simulink model "est_model"  (R2023a)
settings: Solver=VariableStepAuto  StartTime=0.0  StopTime=0.1  FixedStep=Ts  RelTol=1e-6  AbsTol=1e-6
InitFcn:
  | est_model_paras
values from neighbouring files (symbols this model uses):
  Id = 0    [est_model_paras.m]
  Iq = 100    [est_model_paras.m]
  ki = [ki1 ki2]    [est_model_paras.m]    (also in svc_go_init.m = 2.96*Rs/sqrt(2)/N/Ts)
  kid_i = 3*Rs./Npi/Ts/Lq/Iq    [est_model_paras.m]
  kid_p = 3*Lq./Npi/Ts/Lq/Iq    [est_model_paras.m]
  kp = (3*Ld./N/Ts-Rs)/Lq/Iq    [est_model_paras.m]    (also in svc_go_init.m = -0.01944)
  kpi_i = 3*Rs./Npi/Ts    [est_model_paras.m]
  kpi_p = 3*Lq./Npi/Ts    [est_model_paras.m]
  Ld = 0.000891    [est_model_paras.m]    (also in svc_go_init.m = 0.00026)
  Lq = 0.000891    [est_model_paras.m]    (also in svc_go_init.m = 0.000636)
  phi_r = 0.012    [est_model_paras.m]    (also in svc_go_init.m = 0.078)
  Rs = 0.503    [est_model_paras.m]    (also in svc_go_init.m = 0.021)
  Ts = 1/8000    (= 0.000125)    [est_model_paras.m]    (also in svc_go_init.m)
  We = 2*pi*100    (= 628.318530718)    [est_model_paras.m]    (also in svc_go_init.m)
undefined symbols (not defined in the file or in its folder): DiscIntNeverNeededParam, ts
libraries: slpidlib x3
settings Model: Creator=LG-PC  LastModifiedBy=洲
settings SolverCC: AlgebraicLoopSolver=LineSearch
settings DataIOCC: ReturnWorkspaceOutputs=off
settings DebuggingCC: UnconnectedInputMsg=warning  UnconnectedOutputMsg=warning  UnconnectedLineMsg=warning  ArithmeticOperatorsInVariantConditions=warning
settings ModelReferenceCC: EnableRefExpFcnMdlSchedulingChecks=on
settings SFSimCC: SimUseLocalCustomCode=off  CustomCodeUndefinedFunction=UseInterfaceOnly
settings RTWCC: RTWUseLocalCustomCode=off

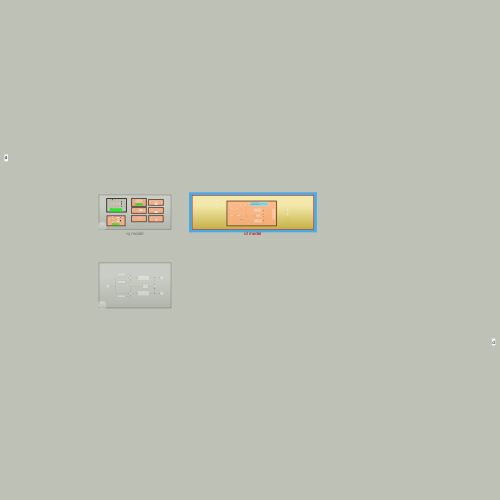
[thumbnail: Simulink's stored preview of the top-level diagram]
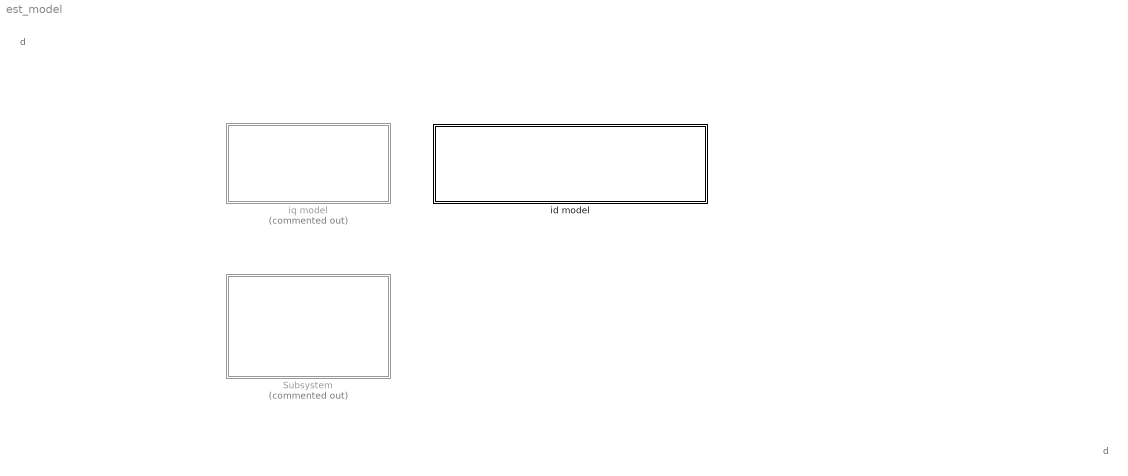
== system est_model ==
  note: d
  note: d
  Subsystem : Subsystem  Commented=on
  id model : Subsystem
  iq model : Subsystem  Commented=on

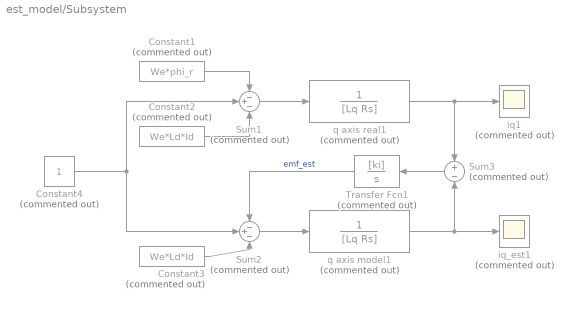
== system est_model/Subsystem ==
  Constant1 : Constant  Commented=on  Value=We*phi_r
  Constant2 : Constant  Commented=on  Value=We*Ld*Id
  Constant3 : Constant  Commented=on  Value=We*Ld*Id
  Constant4 : Constant  Commented=on
  Sum1 : Sum  Commented=on  Inputs=-+-
  Sum2 : Sum  Commented=on  Inputs=-+-
  Sum3 : Sum  Commented=on  Inputs=+-
  Transfer Fcn1 : TransferFcn  Commented=on  Numerator=[ki]  Denominator=[1 0]
  iq1 : Scope  Commented=on
  iq_est1 : Scope  Commented=on
  q axis model1 : TransferFcn  Commented=on  Denominator=[Lq Rs]
  q axis real1 : TransferFcn  Commented=on  Denominator=[Lq Rs]
  wires:
  q axis model1/1 -> iq_est1/1, Sum3/2
  Constant1/1 -> Sum1/1
  q axis real1/1 -> iq1/1, Sum3/1
  Sum3/1 -> Transfer Fcn1/1
  Constant3/1 -> Sum2/3
  Sum2/1 -> q axis model1/1
  Transfer Fcn1/1 -> Sum2/1  "emf_est"
  Constant2/1 -> Sum1/3
  Constant4/1 -> Sum1/2, Sum2/2
  Sum1/1 -> q axis real1/1

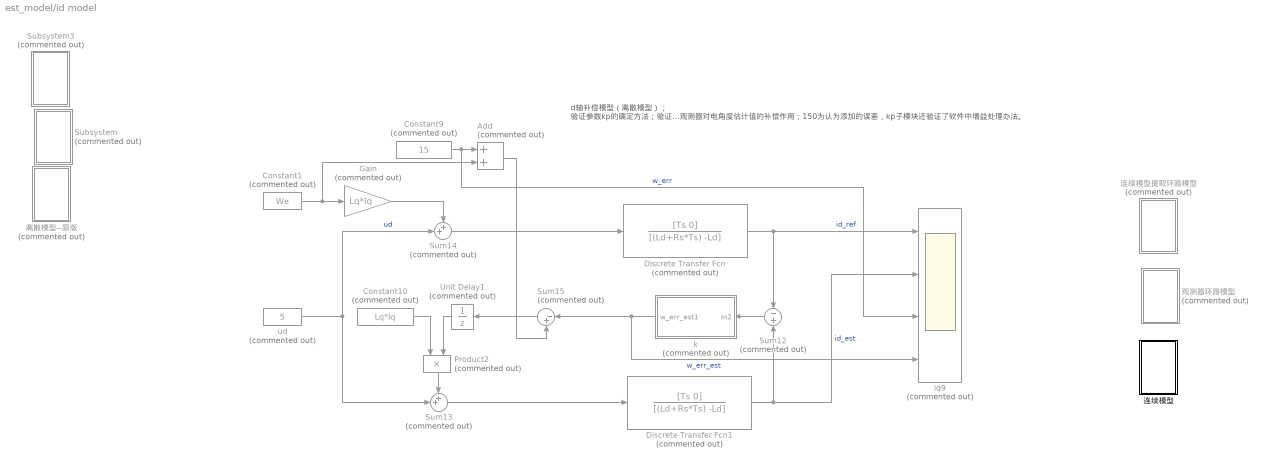
== system est_model/id model ==
  note: d轴补偿模型（离散模型）；
      | 验证参数kp的确定方法；验证观测器对电角度估计值的补偿作用；150为认为添加的误差，kp子模块还验证了软件中增益处理办法。
  Add : Sum  Commented=on
  Constant1 : Constant  Commented=on  Value=We
  Constant10 : Constant  Commented=on  Value=Lq*Iq
  Constant9 : Constant  Commented=on  Value=15
  Discrete Transfer Fcn : DiscreteTransferFcn  Commented=on  Numerator=[Ts 0]  Denominator=[(Ld+Rs*Ts) -Ld]
  Discrete Transfer Fcn1 : DiscreteTransferFcn  Commented=on  Numerator=[Ts 0]  Denominator=[(Ld+Rs*Ts) -Ld]
  Gain : Gain  Commented=on  Gain=Lq*Iq
  Product2 : Product  Commented=on
  Subsystem : Subsystem  Commented=on
  Subsystem3 : Subsystem  Commented=on
  Sum12 : Sum  Commented=on  Inputs=-+
  Sum13 : Sum  Commented=on  Inputs=++|
  Sum14 : Sum  Commented=on  Inputs=++|
  Sum15 : Sum  Commented=on  Inputs=|-+
  Unit Delay1 : UnitDelay  Commented=on  SampleTime=-1  HasFrameUpgradeWarning=on
  iq9 : Scope  Commented=on  NumInputPorts=4
  k : Subsystem  Commented=on
  ud : Constant  Commented=on  Value=5
  离散模型--原版 : Subsystem  Commented=on
  观测器环路模型 : Subsystem  Commented=on
  连续模型 : Subsystem
  连续模型提取环路模型 : Subsystem  Commented=on
  wires:
  ud/1 -> Sum13/2, Sum14/2  "ud"
  Add/1 -> Sum15/2
  Discrete Transfer Fcn/1 -> Sum12/1, iq9/1  "id_ref"
  Sum14/1 -> Discrete Transfer Fcn/1
  Sum15/1 -> Unit Delay1/1
  Product2/1 -> Sum13/1
  Discrete Transfer Fcn1/1 -> iq9/2, Sum12/2  "id_est"
  Unit Delay1/1 -> Product2/2
  Constant10/1 -> Product2/1
  Constant1/1 -> Add/2, Gain/1
  Gain/1 -> Sum14/1
  Sum13/1 -> Discrete Transfer Fcn1/1
  Constant9/1 -> iq9/3, Add/1  "w_err"
  k/1(w_err_est1) -> iq9/4, Sum15/1  "w_err_est"
  Sum12/1 -> k/1(In2)

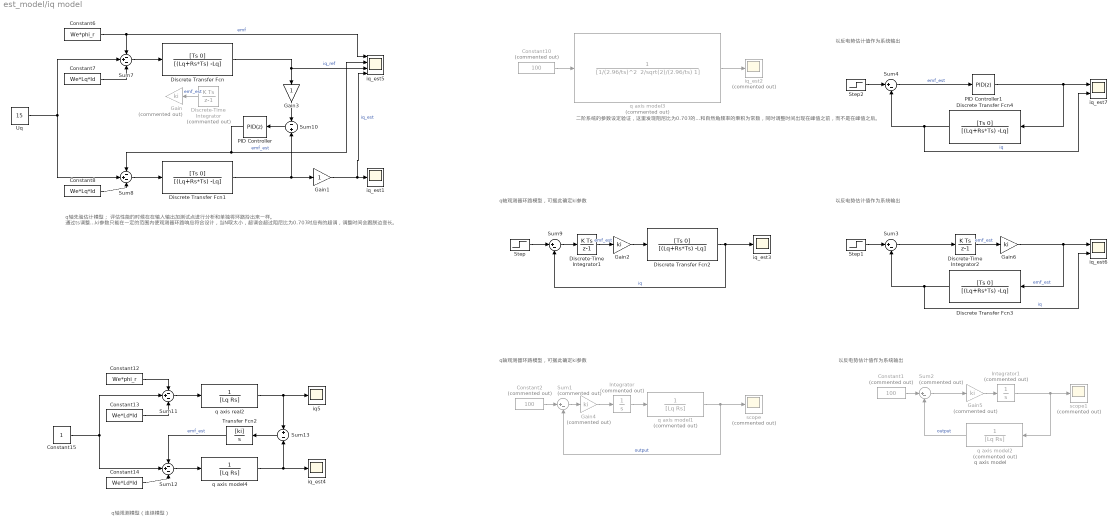
== system est_model/iq model ==
  note: q axis model
  note: q轴观测器环路模型，可据此确定ki参数
  note: 二阶系统的参数设定验证，这里发现阻尼比为0.707的时候，调整时间和自然角频率的乘积为常数，同时调整时间出现在峰值之前，而不是在峰值之后。
  note: q轴观测模型（连续模型）
  note: q轴先验估计模型；
      | 评估性能的时候在在输入输出加测试点进行分析和单独将环路拎出来一样。
      | 通过ts调整ki参数只能在一定的范围内使观测器环路响应符合设计，当N取太小，超调会超过阻尼比为0.707时应有的超调，调整时间会跟朕边变长。
  note: q轴观测器环路模型，可据此确定ki参数
  note: 以反电势估计值作为系统输出
  note: 以反电势估计值作为系统输出
  note: 以反电势估计值作为系统输出
  Constant1 : Constant  Commented=on  Value=100
  Constant10 : Constant  Commented=on  Value=100
  Constant12 : Constant  Value=We*phi_r
  Constant13 : Constant  Value=We*Ld*Id
  Constant14 : Constant  Value=We*Ld*Id
  Constant15 : Constant
  Constant2 : Constant  Commented=on  Value=100
  Constant6 : Constant  Value=We*phi_r
  Constant7 : Constant  Value=We*Lq*Id
  Constant8 : Constant  Value=We*Lq*Id
  Discrete Transfer Fcn{,1..4} (5 alike) : DiscreteTransferFcn  Numerator=[Ts 0]  Denominator=[(Lq+Rs*Ts) -Lq]
  Discrete-Time Integrator : DiscreteIntegrator  Commented=on  SampleTime=-1  ICPrevOutput=DiscIntNeverNeededParam  ICPrevScaledInput=DiscIntNeverNeededParam
  Discrete-Time Integrator1 : DiscreteIntegrator  SampleTime=-1  ICPrevOutput=DiscIntNeverNeededParam  ICPrevScaledInput=DiscIntNeverNeededParam
  Discrete-Time Integrator2 : DiscreteIntegrator  SampleTime=-1  ICPrevOutput=DiscIntNeverNeededParam  ICPrevScaledInput=DiscIntNeverNeededParam
  Gain : Gain  Commented=on  Gain=ki
  Gain1 : Gain
  Gain2 : Gain  Gain=ki
  Gain3 : Gain
  Gain4 : Gain  Commented=on  Gain=ki
  Gain5 : Gain  Commented=on  Gain=ki
  Gain6 : Gain  Gain=ki
  Integrator : Integrator  Commented=on
  Integrator1 : Integrator  Commented=on
  PID Controller : slpidlib/PID Controller  Controller=PID  Form=Parallel  TimeDomain=Discrete-time  UseExternalTs=off  SampleTime=-1  IntegratorMethod=Forward Euler  FilterMethod=Forward Euler  ControllerParametersSource=internal  P=kpi_p  I=kpi_i  UseKiTs=off  D=0  N=100  UseFilter=on  TunerSelectOption=Transfer Function Based (PID Tuner App)  InitialConditionSource=internal  InitialConditionForIntegrator=0  InitialConditionForFilter=0  DifferentiatorICPrevScaledInput=0  ExternalReset=none  TrackingMode=off  Kt=1  LimitOutput=off  SatLimitsSource=internal  UpperSaturationLimit=inf  LowerSaturationLimit=-inf  LinearizeAsGain=on  AntiWindupMode=none  Kb=1  LimitIntegrator=off  UpperIntegratorSaturationLimit=inf  LowerIntegratorSaturationLimit=-inf  POutMin=[]  POutMax=[]  IOutMin=[]  IOutMax=[]  DOutMin=[]  DOutMax=[]  NOutMin=[]  NOutMax=[]  SumOutMin=[]  SumOutMax=[]  SaturationOutMin=[]  SaturationOutMax=[]  PParamMin=[]  PParamMax=[]  IParamMin=[]  IParamMax=[]  DParamMin=[]  DParamMax=[]  NParamMin=[]  NParamMax=[]  KbParamMin=[]  KbParamMax=[]  KtParamMin=[]  KtParamMax=[]  KbOutMin=[]  KbOutMax=[]  KtOutMin=[]  KtOutMax=[]  IntegratorOutMin=[]  IntegratorOutMax=[]  FilterOutMin=[]  FilterOutMax=[]  SumI1OutMin=[]  SumI1OutMax=[]  SumI2OutMin=[]  SumI2OutMax=[]  SumI3OutMin=[]  SumI3OutMax=[]  SumI4OutMin=[]  SumI4OutMax=[]  SumDOutMin=[]  SumDOutMax=[]  DifferentiatorOutMin=[]  DifferentiatorOutMax=[]  FilterDiffOutCoefMin=[]  FilterDiffOutCoefMax=[]  ReciprocalOutMin=[]  ReciprocalOutMax=[]  SumDenOutMin=[]  SumDenOutMax=[]  SumNumOutMin=[]  SumNumOutMax=[]  DivideOutMin=[]  DivideOutMax=[]  UdiffTsProdOutMin=[]  UdiffTsProdOutMax=[]  NTsProdOutMin=[]  NTsProdOutMax=[]  UintegralTsProdOutMin=[]  UintegralTsProdOutMax=[]  UngainTsProdOutMin=[]  UngainTsProdOutMax=[]  ClampingZeroOutDataTypeStr=Inherit: Inherit via back propagation  ClampingZeroOutMin=[]  ClampingZeroOutMax=[]  FilterDenConstantOutDataTypeStr=Inherit: Inherit via back propagation  FilterDenConstantOutMin=[]  FilterDenConstantOutMax=[]  PCopyOutDataTypeStr=Inherit: Inherit via back propagation  PCopyOutMin=[]  PCopyOutMax=[]  NCopyOutDataTypeStr=Inherit: Inherit via back propagation  NCopyOutMin=[]  NCopyOutMax=[]  IntegratorContinuousStateAttributes=''  IntegratorStateMustResolveToSignalObject=off  IntegratorRTWStateStorageClass=Auto  FilterContinuousStateAttributes=''  FilterStateMustResolveToSignalObject=off  FilterRTWStateStorageClass=Auto  ParallelPVariant=InternalParameters  IdealPVariant=Disabled  IVariant=InternalParameters  DVariant=InternalParameters  IntegratorVariant=Discrete  SatVariant=Disabled  AWVariant=Passthrough  PCopyVariant=Disabled  TRVariant=Disabled  FdbkBlocksVariant=Forward  IdealPFdbkVariant=Disabled  SatFdbkVariant=Disabled  DerivativeFilterVariant=ForwardEulerFilter  NVariant=InternalParameters  NCopyVariant=Disabled  FilterICVariant=InternalICsFilter  IntegratorICVariant=InternalICs  ExternalResetVariant=Disabled  TRSumVariant=Passthrough  SumFdbkVariant=Disabled  SumVariant=Sum_PID  TsampFilterVariant=InternalTs  TsampNgainVariant=Passthrough  TsampIntegralVariant=Disabled_SignalSpec  ExternalSaturationOutDataTypeStr=Inherit: Same as second input
  PID Controller1 : slpidlib/PID Controller  Controller=PID  Form=Parallel  TimeDomain=Discrete-time  UseExternalTs=off  SampleTime=-1  IntegratorMethod=Forward Euler  FilterMethod=Forward Euler  ControllerParametersSource=internal  P=1  I=800  UseKiTs=off  D=0  N=100  UseFilter=on  TunerSelectOption=Transfer Function Based (PID Tuner App)  InitialConditionSource=internal  InitialConditionForIntegrator=0  InitialConditionForFilter=0  DifferentiatorICPrevScaledInput=0  ExternalReset=none  TrackingMode=off  Kt=1  LimitOutput=off  SatLimitsSource=internal  UpperSaturationLimit=inf  LowerSaturationLimit=-inf  LinearizeAsGain=on  AntiWindupMode=none  Kb=1  LimitIntegrator=off  UpperIntegratorSaturationLimit=inf  LowerIntegratorSaturationLimit=-inf  POutMin=[]  POutMax=[]  IOutMin=[]  IOutMax=[]  DOutMin=[]  DOutMax=[]  NOutMin=[]  NOutMax=[]  SumOutMin=[]  SumOutMax=[]  SaturationOutMin=[]  SaturationOutMax=[]  PParamMin=[]  PParamMax=[]  IParamMin=[]  IParamMax=[]  DParamMin=[]  DParamMax=[]  NParamMin=[]  NParamMax=[]  KbParamMin=[]  KbParamMax=[]  KtParamMin=[]  KtParamMax=[]  KbOutMin=[]  KbOutMax=[]  KtOutMin=[]  KtOutMax=[]  IntegratorOutMin=[]  IntegratorOutMax=[]  FilterOutMin=[]  FilterOutMax=[]  SumI1OutMin=[]  SumI1OutMax=[]  SumI2OutMin=[]  SumI2OutMax=[]  SumI3OutMin=[]  SumI3OutMax=[]  SumI4OutMin=[]  SumI4OutMax=[]  SumDOutMin=[]  SumDOutMax=[]  DifferentiatorOutMin=[]  DifferentiatorOutMax=[]  FilterDiffOutCoefMin=[]  FilterDiffOutCoefMax=[]  ReciprocalOutMin=[]  ReciprocalOutMax=[]  SumDenOutMin=[]  SumDenOutMax=[]  SumNumOutMin=[]  SumNumOutMax=[]  DivideOutMin=[]  DivideOutMax=[]  UdiffTsProdOutMin=[]  UdiffTsProdOutMax=[]  NTsProdOutMin=[]  NTsProdOutMax=[]  UintegralTsProdOutMin=[]  UintegralTsProdOutMax=[]  UngainTsProdOutMin=[]  UngainTsProdOutMax=[]  ClampingZeroOutDataTypeStr=Inherit: Inherit via back propagation  ClampingZeroOutMin=[]  ClampingZeroOutMax=[]  FilterDenConstantOutDataTypeStr=Inherit: Inherit via back propagation  FilterDenConstantOutMin=[]  FilterDenConstantOutMax=[]  PCopyOutDataTypeStr=Inherit: Inherit via back propagation  PCopyOutMin=[]  PCopyOutMax=[]  NCopyOutDataTypeStr=Inherit: Inherit via back propagation  NCopyOutMin=[]  NCopyOutMax=[]  IntegratorContinuousStateAttributes=''  IntegratorStateMustResolveToSignalObject=off  IntegratorRTWStateStorageClass=Auto  FilterContinuousStateAttributes=''  FilterStateMustResolveToSignalObject=off  FilterRTWStateStorageClass=Auto  ParallelPVariant=InternalParameters  IdealPVariant=Disabled  IVariant=InternalParameters  DVariant=InternalParameters  IntegratorVariant=Discrete  SatVariant=Disabled  AWVariant=Passthrough  PCopyVariant=Disabled  TRVariant=Disabled  FdbkBlocksVariant=Forward  IdealPFdbkVariant=Disabled  SatFdbkVariant=Disabled  DerivativeFilterVariant=ForwardEulerFilter  NVariant=InternalParameters  NCopyVariant=Disabled  FilterICVariant=InternalICsFilter  IntegratorICVariant=InternalICs  ExternalResetVariant=Disabled  TRSumVariant=Passthrough  SumFdbkVariant=Disabled  SumVariant=Sum_PID  TsampFilterVariant=InternalTs  TsampNgainVariant=Passthrough  TsampIntegralVariant=Disabled_SignalSpec  ExternalSaturationOutDataTypeStr=Inherit: Same as second input
  Step : Step  Time=0.02  After=100  SampleTime=0
  Step1 : Step  Time=0.02  After=100  SampleTime=0
  Step2 : Step  Time=0.02  After=100  SampleTime=0
  Sum1 : Sum  Commented=on  Inputs=|+-
  Sum10 : Sum  Inputs=-+
  Sum{7..8,11..12} (4 alike) : Sum  Inputs=-+-
  Sum13 : Sum  Inputs=+-
  Sum2 : Sum  Commented=on  Inputs=|+-
  Sum3 : Sum  Inputs=|+-
  Sum4 : Sum  Inputs=|+-
  Sum9 : Sum  Inputs=|+-
  Transfer Fcn2 : TransferFcn  Numerator=[ki]  Denominator=[1 0]
  Uq : Constant  Value=15
  iq5 : Scope
  iq_est1 : Scope
  iq_est2 : Scope  Commented=on
  iq_est3 : Scope
  iq_est4 : Scope
  iq_est5 : Scope  NumInputPorts=4
  iq_est6 : Scope  NumInputPorts=2
  iq_est7 : Scope  NumInputPorts=2
  q axis model1 : TransferFcn  Commented=on  Denominator=[Lq Rs]
  q axis model2 : TransferFcn  Commented=on  Denominator=[Lq Rs]
  q axis model3 : TransferFcn  Commented=on  Denominator="[1/(2.96/ts)^2  2/sqrt(2)/(2.96/ts) 1]"
  q axis model4 : TransferFcn  Denominator=[Lq Rs]
  q axis real2 : TransferFcn  Denominator=[Lq Rs]
  scope : Scope  Commented=on
  scope1 : Scope  Commented=on
  wires:
  Discrete-Time Integrator/1 -> Gain/1  "emf_est"
  Constant6/1 -> Sum7/1, iq_est5/1  "emf"
  Uq/1 -> Sum7/2, Sum8/2
  Discrete Transfer Fcn1/1 -> Gain1/1, Sum10/2
  Sum7/1 -> Discrete Transfer Fcn/1
  Constant7/1 -> Sum7/3
  Sum8/1 -> Discrete Transfer Fcn1/1
  Constant8/1 -> Sum8/3
  q axis model3/1 -> iq_est2/1
  Constant10/1 -> q axis model3/1
  Gain1/1 -> iq_est5/4, iq_est1/1  "iq_est"
  Discrete Transfer Fcn2/1 -> iq_est3/1, Sum9/2  "iq"
  Sum9/1 -> Discrete-Time Integrator1/1
  Gain3/1 -> Sum10/1
  Step/1 -> Sum9/1
  Discrete Transfer Fcn/1 -> iq_est5/3, Gain3/1  "iq_ref"
  q axis model4/1 -> iq_est4/1, Sum13/2
  Constant12/1 -> Sum11/1
  q axis real2/1 -> iq5/1, Sum13/1
  Sum13/1 -> Transfer Fcn2/1
  Constant14/1 -> Sum12/3
  Sum12/1 -> q axis model4/1
  Transfer Fcn2/1 -> Sum12/1  "emf_est"
  Constant13/1 -> Sum11/3
  Constant15/1 -> Sum11/2, Sum12/2
  Sum11/1 -> q axis real2/1
  Gain2/1 -> Discrete Transfer Fcn2/1
  Gain4/1 -> Integrator/1
  Integrator/1 -> q axis model1/1
  Constant2/1 -> Sum1/1
  Sum1/1 -> Gain4/1
  q axis model1/1 -> scope/1, Sum1/2  "output"
  Discrete-Time Integrator1/1 -> Gain2/1  "emf_est"
  Sum10/1 -> PID Controller/1
  Gain6/1 -> iq_est6/1, Discrete Transfer Fcn3/1  "emf_est"
  Discrete-Time Integrator2/1 -> Gain6/1  "emf_est"
  Sum3/1 -> Discrete-Time Integrator2/1
  Discrete Transfer Fcn3/1 -> iq_est6/2, Sum3/2  "iq"
  Step1/1 -> Sum3/1
  q axis model2/1 -> Sum2/2  "output"
  Sum2/1 -> Gain5/1
  Constant1/1 -> Sum2/1
  Integrator1/1 -> scope1/1, q axis model2/1
  Gain5/1 -> Integrator1/1
  Discrete Transfer Fcn4/1 -> iq_est7/2, Sum4/2  "iq"
  Sum4/1 -> PID Controller1/1  "emf_est"
  Step2/1 -> Sum4/1
  PID Controller1/1 -> iq_est7/1, Discrete Transfer Fcn4/1
  PID Controller/1 -> iq_est5/2, Sum8/1  "emf_est"

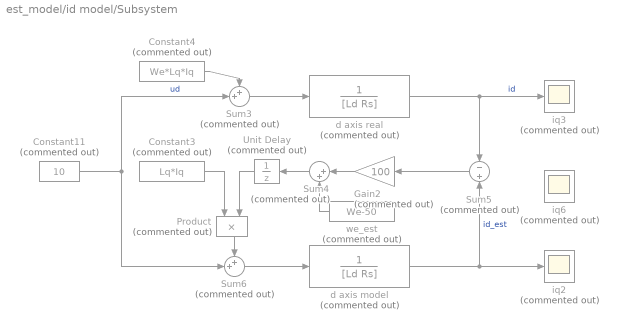
== system est_model/id model/Subsystem ==
  Constant11 : Constant  Commented=on  Value=10
  Constant3 : Constant  Commented=on  Value=Lq*Iq
  Constant4 : Constant  Commented=on  Value=We*Lq*Iq
  Gain2 : Gain  Commented=on  Gain=100
  Product : Product  Commented=on
  Sum3 : Sum  Commented=on  Inputs=++|
  Sum4 : Sum  Commented=on  Inputs=|++
  Sum5 : Sum  Commented=on  Inputs=-+
  Sum6 : Sum  Commented=on  Inputs=++|
  Unit Delay : UnitDelay  Commented=on  SampleTime=-1  HasFrameUpgradeWarning=on
  d axis model : TransferFcn  Commented=on  Denominator=[Ld Rs]
  d axis real : TransferFcn  Commented=on  Denominator=[Ld Rs]
  iq2 : Scope  Commented=on
  iq3 : Scope  Commented=on
  iq6 : Scope  Commented=on
  we_est : Constant  Commented=on  Value=We-50
  wires:
  Sum3/1 -> d axis real/1
  Sum4/1 -> Unit Delay/1
  Sum5/1 -> Gain2/1
  d axis real/1 -> iq3/1, Sum5/1  "id"
  Constant11/1 -> Sum3/2, Sum6/2  "ud"
  Constant4/1 -> Sum3/1
  Product/1 -> Sum6/1
  Constant3/1 -> Product/1
  d axis model/1 -> iq2/1, Sum5/2  "id_est"
  Gain2/1 -> Sum4/1
  Unit Delay/1 -> Product/2
  we_est/1 -> Sum4/2
  Sum6/1 -> d axis model/1
  ? -> iq6/1

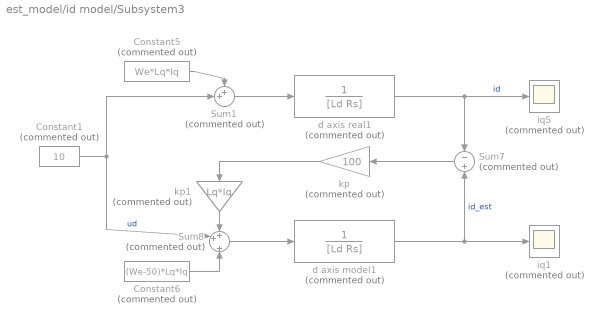
== system est_model/id model/Subsystem3 ==
  Constant1 : Constant  Commented=on  Value=10
  Constant5 : Constant  Commented=on  Value=We*Lq*Iq
  Constant6 : Constant  Commented=on  Value=(We-50)*Lq*Iq
  Sum1 : Sum  Commented=on  Inputs=++|
  Sum7 : Sum  Commented=on  Inputs=-+
  Sum8 : Sum  Commented=on  Inputs=++|+
  d axis model1 : TransferFcn  Commented=on  Denominator=[Ld Rs]
  d axis real1 : TransferFcn  Commented=on  Denominator=[Ld Rs]
  iq1 : Scope  Commented=on
  iq5 : Scope  Commented=on
  kp : Gain  Commented=on  Gain=100
  kp1 : Gain  Commented=on  Gain=Lq*Iq
  wires:
  Sum1/1 -> d axis real1/1
  Constant6/1 -> Sum8/3
  kp/1 -> kp1/1
  d axis real1/1 -> iq5/1, Sum7/1  "id"
  d axis model1/1 -> iq1/1, Sum7/2  "id_est"
  Constant1/1 -> Sum1/2, Sum8/2  "ud"
  Sum8/1 -> d axis model1/1
  Sum7/1 -> kp/1
  kp1/1 -> Sum8/1
  Constant5/1 -> Sum1/1

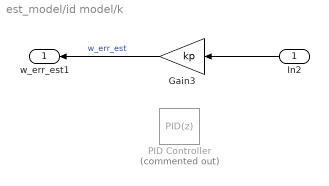
== system est_model/id model/k ==
  In2 : Inport
  Gain3 : Gain  Gain=kp
  PID Controller : slpidlib/PID Controller  Commented=on  Controller=PID  Form=Parallel  TimeDomain=Discrete-time  UseExternalTs=off  SampleTime=-1  IntegratorMethod=Forward Euler  FilterMethod=Forward Euler  ControllerParametersSource=internal  P=kid_p  I=kid_i  UseKiTs=off  D=0  N=100  UseFilter=on  TunerSelectOption=Transfer Function Based (PID Tuner App)  InitialConditionSource=internal  InitialConditionForIntegrator=0  InitialConditionForFilter=0  DifferentiatorICPrevScaledInput=0  ExternalReset=none  TrackingMode=off  Kt=1  LimitOutput=off  SatLimitsSource=internal  UpperSaturationLimit=inf  LowerSaturationLimit=-inf  LinearizeAsGain=on  AntiWindupMode=none  Kb=1  LimitIntegrator=off  UpperIntegratorSaturationLimit=inf  LowerIntegratorSaturationLimit=-inf  POutMin=[]  POutMax=[]  IOutMin=[]  IOutMax=[]  DOutMin=[]  DOutMax=[]  NOutMin=[]  NOutMax=[]  SumOutMin=[]  SumOutMax=[]  SaturationOutMin=[]  SaturationOutMax=[]  PParamMin=[]  PParamMax=[]  IParamMin=[]  IParamMax=[]  DParamMin=[]  DParamMax=[]  NParamMin=[]  NParamMax=[]  KbParamMin=[]  KbParamMax=[]  KtParamMin=[]  KtParamMax=[]  KbOutMin=[]  KbOutMax=[]  KtOutMin=[]  KtOutMax=[]  IntegratorOutMin=[]  IntegratorOutMax=[]  FilterOutMin=[]  FilterOutMax=[]  SumI1OutMin=[]  SumI1OutMax=[]  SumI2OutMin=[]  SumI2OutMax=[]  SumI3OutMin=[]  SumI3OutMax=[]  SumI4OutMin=[]  SumI4OutMax=[]  SumDOutMin=[]  SumDOutMax=[]  DifferentiatorOutMin=[]  DifferentiatorOutMax=[]  FilterDiffOutCoefMin=[]  FilterDiffOutCoefMax=[]  ReciprocalOutMin=[]  ReciprocalOutMax=[]  SumDenOutMin=[]  SumDenOutMax=[]  SumNumOutMin=[]  SumNumOutMax=[]  DivideOutMin=[]  DivideOutMax=[]  UdiffTsProdOutMin=[]  UdiffTsProdOutMax=[]  NTsProdOutMin=[]  NTsProdOutMax=[]  UintegralTsProdOutMin=[]  UintegralTsProdOutMax=[]  UngainTsProdOutMin=[]  UngainTsProdOutMax=[]  ClampingZeroOutDataTypeStr=Inherit: Inherit via back propagation  ClampingZeroOutMin=[]  ClampingZeroOutMax=[]  FilterDenConstantOutDataTypeStr=Inherit: Inherit via back propagation  FilterDenConstantOutMin=[]  FilterDenConstantOutMax=[]  PCopyOutDataTypeStr=Inherit: Inherit via back propagation  PCopyOutMin=[]  PCopyOutMax=[]  NCopyOutDataTypeStr=Inherit: Inherit via back propagation  NCopyOutMin=[]  NCopyOutMax=[]  IntegratorContinuousStateAttributes=''  IntegratorStateMustResolveToSignalObject=off  IntegratorRTWStateStorageClass=Auto  FilterContinuousStateAttributes=''  FilterStateMustResolveToSignalObject=off  FilterRTWStateStorageClass=Auto  ParallelPVariant=InternalParameters  IdealPVariant=Disabled  IVariant=InternalParameters  DVariant=InternalParameters  IntegratorVariant=Discrete  SatVariant=Disabled  AWVariant=Passthrough  PCopyVariant=Disabled  TRVariant=Disabled  FdbkBlocksVariant=Forward  IdealPFdbkVariant=Disabled  SatFdbkVariant=Disabled  DerivativeFilterVariant=ForwardEulerFilter  NVariant=InternalParameters  NCopyVariant=Disabled  FilterICVariant=InternalICsFilter  IntegratorICVariant=InternalICs  ExternalResetVariant=Disabled  TRSumVariant=Passthrough  SumFdbkVariant=Disabled  SumVariant=Sum_PID  TsampFilterVariant=InternalTs  TsampNgainVariant=Passthrough  TsampIntegralVariant=Disabled_SignalSpec  ExternalSaturationOutDataTypeStr=Inherit: Same as second input
  w_err_est1 : Outport  VectorParamsAs1DForOutWhenUnconnected=off
  wires:
  In2/1 -> Gain3/1
  Gain3/1 -> w_err_est1/1  "w_err_est"

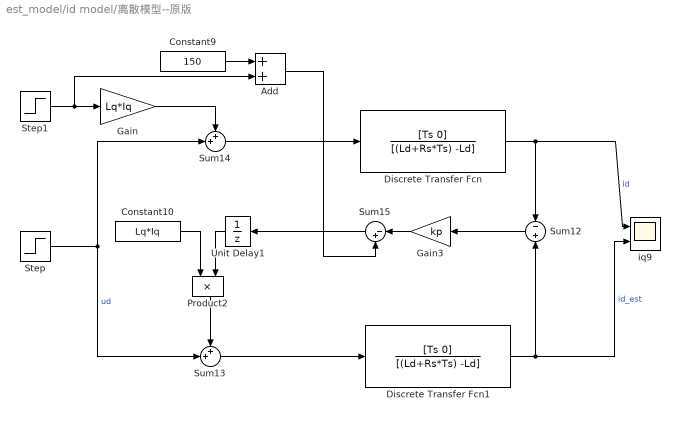
== system est_model/id model/离散模型--原版 ==
  Add : Sum
  Constant10 : Constant  Value=Lq*Iq
  Constant9 : Constant  Value=150
  Discrete Transfer Fcn : DiscreteTransferFcn  Numerator=[Ts 0]  Denominator=[(Ld+Rs*Ts) -Ld]
  Discrete Transfer Fcn1 : DiscreteTransferFcn  Numerator=[Ts 0]  Denominator=[(Ld+Rs*Ts) -Ld]
  Gain : Gain  Gain=Lq*Iq
  Gain3 : Gain  Gain=kp
  Product2 : Product
  Step : Step  Time=0.02  After=10  SampleTime=0
  Step1 : Step  Time=0.02  After=We  SampleTime=0
  Sum12 : Sum  Inputs=-+
  Sum13 : Sum  Inputs=++|
  Sum14 : Sum  Inputs=++|
  Sum15 : Sum  Inputs=|-+
  Unit Delay1 : UnitDelay  SampleTime=-1  HasFrameUpgradeWarning=on
  iq9 : Scope  NumInputPorts=2
  wires:
  Sum13/1 -> Discrete Transfer Fcn1/1
  Gain3/1 -> Sum15/1
  Gain/1 -> Sum14/1
  Unit Delay1/1 -> Product2/2
  Constant9/1 -> Add/1
  Constant10/1 -> Product2/1
  Step1/1 -> Add/2, Gain/1
  Sum12/1 -> Gain3/1
  Discrete Transfer Fcn1/1 -> Sum12/2, iq9/2  "id_est"
  Product2/1 -> Sum13/1
  Sum15/1 -> Unit Delay1/1
  Sum14/1 -> Discrete Transfer Fcn/1
  Step/1 -> Sum13/2, Sum14/2  "ud"
  Discrete Transfer Fcn/1 -> Sum12/1, iq9/1  "id"
  Add/1 -> Sum15/2

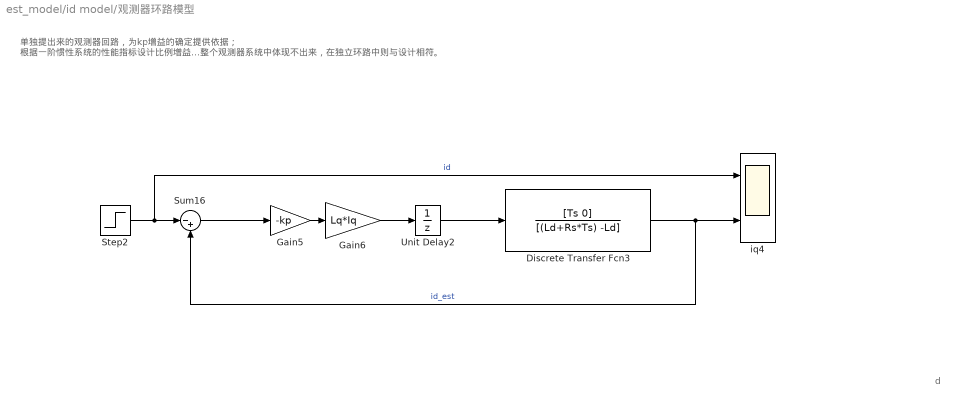
== system est_model/id model/观测器环路模型 ==
  note: d
  note: 单独提出来的观测器回路，为kp增益的确定提供依据；
      | 根据一阶惯性系统的性能指标设计比例增益，设计结果在整个观测器系统中体现不出来，在独立环路中则与设计相符。
  Discrete Transfer Fcn3 : DiscreteTransferFcn  Numerator=[Ts 0]  Denominator=[(Ld+Rs*Ts) -Ld]
  Gain5 : Gain  Gain=-kp
  Gain6 : Gain  Gain=Lq*Iq
  Step2 : Step  Time=0.02  After=100  SampleTime=0
  Sum16 : Sum  Inputs=|-+
  Unit Delay2 : UnitDelay  SampleTime=-1  HasFrameUpgradeWarning=on
  iq4 : Scope  NumInputPorts=2
  wires:
  Gain5/1 -> Gain6/1
  Step2/1 -> iq4/1, Sum16/1  "id"
  Discrete Transfer Fcn3/1 -> Sum16/2, iq4/2  "id_est"
  Sum16/1 -> Gain5/1
  Unit Delay2/1 -> Discrete Transfer Fcn3/1
  Gain6/1 -> Unit Delay2/1

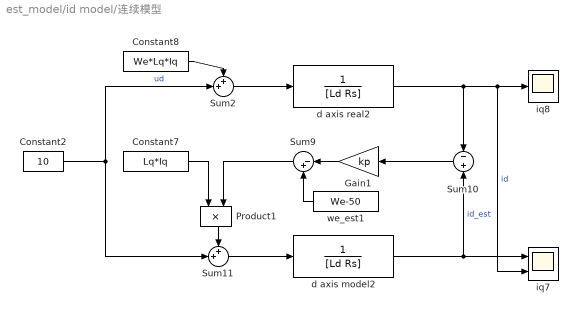
== system est_model/id model/连续模型 ==
  Constant2 : Constant  Value=10
  Constant7 : Constant  Value=Lq*Iq
  Constant8 : Constant  Value=We*Lq*Iq
  Gain1 : Gain  Gain=kp
  Product1 : Product
  Sum10 : Sum  Inputs=-+
  Sum11 : Sum  Inputs=++|
  Sum2 : Sum  Inputs=++|
  Sum9 : Sum  Inputs=|-+
  d axis model2 : TransferFcn  Denominator=[Ld Rs]
  d axis real2 : TransferFcn  Denominator=[Ld Rs]
  iq7 : Scope  NumInputPorts=2
  iq8 : Scope
  we_est1 : Constant  Value=We-50
  wires:
  Gain1/1 -> Sum9/1
  Sum9/1 -> Product1/2
  d axis real2/1 -> iq7/2, iq8/1, Sum10/1  "id"
  d axis model2/1 -> iq7/1, Sum10/2  "id_est"
  Sum11/1 -> d axis model2/1
  we_est1/1 -> Sum9/2
  Constant7/1 -> Product1/1
  Sum10/1 -> Gain1/1
  Product1/1 -> Sum11/1
  Constant8/1 -> Sum2/1
  Constant2/1 -> Sum2/2, Sum11/2  "ud"
  Sum2/1 -> d axis real2/1

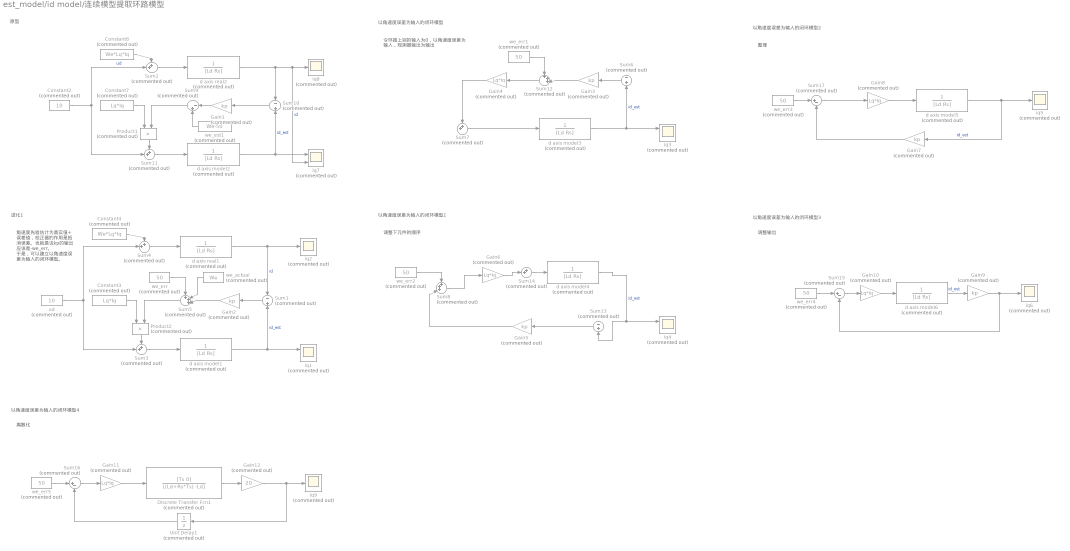
== system est_model/id model/连续模型提取环路模型 ==
  note: 角速度先验估计为真实值+
      | 误差值，校正器的作用是抵
      | 消误差。也就是说kp的输出
      | 应该是-we_err。
      | 于是，可以建立以角速度误
      | 差为输入的闭环模型。
  note: 进化1
  note: 原型
  note: 以角速度误差为输入的闭环模型
  note: 令环路上别的输入为0，以角速度误差为
      | 输入，观测器输出为输出
  note: 调整下元件的顺序
  note: 以角速度误差为输入的闭环模型1
  note: 整理
  note: 以角速度误差为输入的闭环模型2
  note: 调整输出
  note: 以角速度误差为输入的闭环模型3
  note: 以角速度误差为输入的闭环模型4
  note: 离散化
  Constant2 : Constant  Commented=on  Value=10
  Constant3 : Constant  Commented=on  Value=Lq*Iq
  Constant4 : Constant  Commented=on  Value=We*Lq*Iq
  Constant7 : Constant  Commented=on  Value=Lq*Iq
  Constant8 : Constant  Commented=on  Value=We*Lq*Iq
  Discrete Transfer Fcn1 : DiscreteTransferFcn  Commented=on  Numerator=[Ts 0]  Denominator=[(Ld+Rs*Ts) -Ld]
  Gain{1..3,5,7,9} (6 alike) : Gain  Commented=on  Gain=kp
  Gain{4,6,8,10..11} (5 alike) : Gain  Commented=on  Gain=Lq*Iq
  Gain12 : Gain  Commented=on  Gain=20
  Product1 : Product  Commented=on
  Product2 : Product  Commented=on
  Sum{1,6,10,13} (4 alike) : Sum  Commented=on  Inputs=-+
  Sum{2..4,7,11,14} (6 alike) : Sum  Commented=on  Inputs=++|
  Sum12 : Sum  Commented=on  Inputs=+++|
  Sum15 : Sum  Commented=on  Inputs=|+-
  Sum16 : Sum  Commented=on  Inputs=|+-
  Sum17 : Sum  Commented=on  Inputs=|+-
  Sum5 : Sum  Commented=on  Inputs=+++|
  Sum8 : Sum  Commented=on  Inputs=+++|
  Sum9 : Sum  Commented=on  Inputs=|-+
  Unit Delay1 : UnitDelay  Commented=on  SampleTime=-1  HasFrameUpgradeWarning=on
  d axis model{1..6} (6 alike) : TransferFcn  Commented=on  Denominator=[Ld Rs]
  d axis real1 : TransferFcn  Commented=on  Denominator=[Ld Rs]
  d axis real2 : TransferFcn  Commented=on  Denominator=[Ld Rs]
  iq{1,3..4,7} (4 alike) : Scope  Commented=on  NumInputPorts=2
  iq{2,5..6,8..9} (5 alike) : Scope  Commented=on
  ud : Constant  Commented=on  Value=10
  we_actual : Constant  Commented=on  Value=We
  we_err{,1..5} (6 alike) : Constant  Commented=on  Value=50
  we_est1 : Constant  Commented=on  Value=We-50
  wires:
  Constant2/1 -> Sum11/2, Sum2/2  "ud"
  Sum2/1 -> d axis real2/1
  Sum11/1 -> d axis model2/1
  Product1/1 -> Sum11/1
  d axis real2/1 -> Sum10/1, iq8/1, iq7/2  "id"
  Constant8/1 -> Sum2/1
  we_est1/1 -> Sum9/2
  Gain1/1 -> Sum9/1
  Sum9/1 -> Product1/2
  Constant7/1 -> Product1/1
  d axis model2/1 -> Sum10/2, iq7/1  "id_est"
  Sum10/1 -> Gain1/1
  Constant4/1 -> Sum4/1
  Constant3/1 -> Product2/1
  d axis real1/1 -> iq2/1, Sum1/1  "id"
  d axis model1/1 -> iq1/1, Sum1/2  "id_est"
  Product2/1 -> Sum3/1
  Sum1/1 -> Gain2/1
  Sum5/1 -> Product2/2
  Sum3/1 -> d axis model1/1
  Sum4/1 -> d axis real1/1
  ud/1 -> Sum4/2, Sum3/2
  Gain2/1 -> Sum5/3
  we_actual/1 -> Sum5/2
  we_err/1 -> Sum5/1
  we_err1/1 -> Sum12/1
  Sum7/1 -> d axis model3/1
  Sum12/1 -> Gain4/1
  d axis model3/1 -> iq3/1, Sum6/2  "id_est"
  Sum6/1 -> Gain3/1
  Gain3/1 -> Sum12/3
  Gain4/1 -> Sum7/1
  Gain6/1 -> Sum14/2
  Sum13/1 -> Gain5/1
  d axis model4/1 -> iq4/1, Sum13/2  "id_est"
  Sum8/1 -> Gain6/1
  Gain5/1 -> Sum8/3
  we_err2/1 -> Sum8/1
  Sum14/1 -> d axis model4/1
  Sum17/1 -> Gain8/1
  we_err3/1 -> Sum17/1
  Gain7/1 -> Sum17/2
  Gain8/1 -> d axis model5/1
  d axis model5/1 -> Gain7/1, iq5/1  "id_est"
  Sum15/1 -> Gain10/1
  Gain9/1 -> iq6/1, Sum15/2
  Gain10/1 -> d axis model6/1
  d axis model6/1 -> Gain9/1  "id_est"
  we_err4/1 -> Sum15/1
  Gain12/1 -> iq9/1, Unit Delay1/1
  Gain11/1 -> Discrete Transfer Fcn1/1
  Sum16/1 -> Gain11/1
  we_err5/1 -> Sum16/1
  Discrete Transfer Fcn1/1 -> Gain12/1
  Unit Delay1/1 -> Sum16/2
